simulink model "Luanvancu"  (R2018a)
settings: Solver=ode5  StartTime=0.0  StopTime=100  FixedStep=0.05  RelTol=1e-3
settings Model: PacingRate=100  Creator=Hungs  LastModifiedBy=Hungs

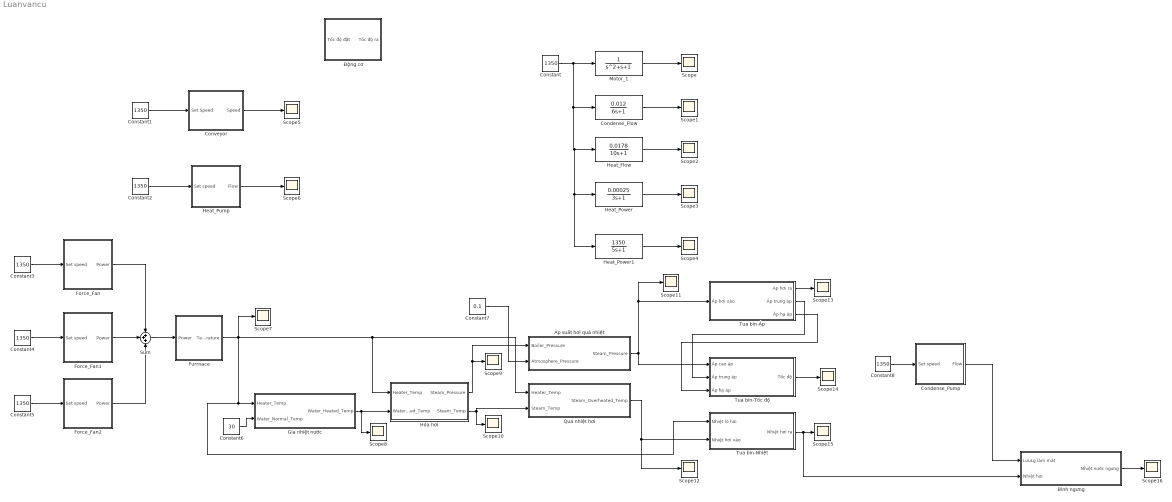
== system Luanvancu ==
  Bình ngưng : Subsystem
  Condense_Flow : TransferFcn  Numerator=[0.012]  Denominator=[6 1]
  Condense_Pump : Subsystem
      mask Display: image('C:\Program Files\MATLAB\ThermalElectricity\Maskicon\Pump.png');
  Constant{,1..5,8} (7 alike) : Constant  Value=1350
  Constant6 : Constant  Value=30
  Constant7 : Constant  Value=0.1
  Conveyor : Subsystem
      mask Display: image('C:\Program Files\MATLAB\ThermalElectricity\Maskicon\conveyor.png');
  Force_Fan : Subsystem
      mask Display: image('C:\Program Files\MATLAB\ThermalElectricity\Maskicon\Fan.png');
  Force_Fan1 : Subsystem
      mask Display: image('C:\Program Files\MATLAB\ThermalElectricity\Maskicon\Fan.png');
  Force_Fan2 : Subsystem
      mask Display: image('C:\Program Files\MATLAB\ThermalElectricity\Maskicon\Fan.png');
  Furrnace : Subsystem
      mask Display: image('C:\Program Files\MATLAB\ThermalElectricity\Maskicon\Furnace.png');
  Gia nhiệt nước : Subsystem
  Heat_Flow : TransferFcn  Numerator=[0.0178]  Denominator=[10 1]
  Heat_Power : TransferFcn  Numerator=[0.00025]  Denominator=[3 1]
  Heat_Power1 : TransferFcn  Numerator=[1350]  Denominator=[5 1]
  Heat_Pump : Subsystem
      mask Display: image('C:\Program Files\MATLAB\ThermalElectricity\Maskicon\Pump.png');
  Hóa hơi : Subsystem
  Motor_1 : TransferFcn  Denominator=[1 1 1]
  Quá nhiệt hơi : Subsystem
  Scope{,1..16} (17 alike) : Scope
  Sum : Sum  Inputs=+++
  Tua bin-Nhiệt : Subsystem
  Tua bin-Tốc độ : Subsystem
  Tua bin-Áp : Subsystem
  Áp suất hơi quá nhiệt : Subsystem
  Động cơ : Subsystem
  wires:
  Motor_1/1 -> Scope/1
  Condense_Flow/1 -> Scope1/1
  Heat_Flow/1 -> Scope2/1
  Constant/1 -> Heat_Power1/1, Heat_Power/1, Heat_Flow/1, Condense_Flow/1, Motor_1/1
  Heat_Power/1 -> Scope3/1
  Heat_Power1/1 -> Scope4/1
  Constant1/1 -> Conveyor/1(Set Speed)
  Conveyor/1(Speed) -> Scope5/1
  Constant2/1 -> Heat_Pump/1(Set speed)
  Heat_Pump/1(Flow) -> Scope6/1
  Force_Fan/1(Power) -> Sum/1
  Constant3/1 -> Force_Fan/1(Set speed)
  Furrnace/1(Temperature) -> Quá nhiệt hơi/1(Heater_Temp), Hóa hơi/1(Heater_Temp), Gia nhiệt nước/1(Heater_Temp), Tua bin-Nhiệt/1(Nhiệt lò hơi), Scope7/1
  Constant4/1 -> Force_Fan1/1(Set speed)
  Force_Fan2/1(Power) -> Sum/3
  Constant5/1 -> Force_Fan2/1(Set speed)
  Sum/1 -> Furrnace/1(Power)
  Force_Fan1/1(Power) -> Sum/2
  Constant6/1 -> Gia nhiệt nước/2(Water_Normal_Temp)
  Gia nhiệt nước/1(Water_Heated_Temp) -> Scope8/1, Hóa hơi/2(Water_Heated_Temp)
  Hóa hơi/1(Steam_Pressure) -> Áp suất hơi quá nhiệt/1(Boiler_Pressure), Scope9/1
  Hóa hơi/2(Steam_Temp) -> Quá nhiệt hơi/2(Steam_Temp), Scope10/1
  Áp suất hơi quá nhiệt/1(Steam_Pressure) -> Tua bin-Tốc độ/1(Áp cao áp), Tua bin-Áp/1(Áp hơi vào), Scope11/1
  Quá nhiệt hơi/1(Steam_Overheated_Temp) -> Tua bin-Nhiệt/2(Nhiệt hơi vào), Scope12/1
  Constant7/1 -> Áp suất hơi quá nhiệt/2(Atmosphere_Pressure)
  Tua bin-Áp/3(Áp hạ áp) -> Tua bin-Tốc độ/3(Áp hạ áp)
  Tua bin-Áp/2(Áp trung áp) -> Tua bin-Tốc độ/2(Áp trung áp)
  Tua bin-Áp/1(Áp hơi ra) -> Scope13/1
  Tua bin-Tốc độ/1(Tốc độ) -> Scope14/1
  Tua bin-Nhiệt/1(Nhiệt hơi ra) -> Bình ngưng/2(Nhiệt hơi), Scope15/1
  Constant8/1 -> Condense_Pump/1(Set speed)
  Condense_Pump/1(Flow) -> Bình ngưng/1(LưuLg làm mát)
  Bình ngưng/1(Nhiệt nước ngưng) -> Scope16/1

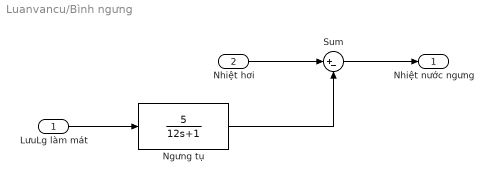
== system Luanvancu/Bình ngưng ==
  LưuLg làm mát : Inport
  Nhiệt hơi : Inport  Port=2
  Ngưng tụ : TransferFcn  Numerator=[5]  Denominator=[12 1]
  Sum : Sum  Inputs=|+-
  Nhiệt nước ngưng : Outport
  wires:
  Sum/1 -> Nhiệt nước ngưng/1
  Ngưng tụ/1 -> Sum/2
  Nhiệt hơi/1 -> Sum/1
  LưuLg làm mát/1 -> Ngưng tụ/1

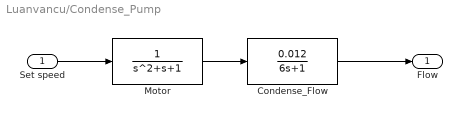
== system Luanvancu/Condense_Pump ==
  Set speed : Inport
  Condense_Flow : TransferFcn  Numerator=[0.012]  Denominator=[6 1]
  Motor : TransferFcn  Denominator=[1 1 1]
  Flow : Outport
  wires:
  Motor/1 -> Condense_Flow/1
  Set speed/1 -> Motor/1
  Condense_Flow/1 -> Flow/1

== system Luanvancu/Conveyor ==
  Set Speed : Inport
  Motor_1 : TransferFcn  Denominator=[1 1 1]
  Speed : Outport
  wires:
  Set Speed/1 -> Motor_1/1
  Motor_1/1 -> Speed/1

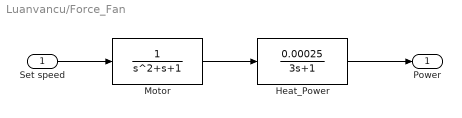
== system Luanvancu/Force_Fan ==
  Set speed : Inport
  Heat_Power : TransferFcn  Numerator=[0.00025]  Denominator=[3 1]
  Motor : TransferFcn  Denominator=[1 1 1]
  Power : Outport
  wires:
  Motor/1 -> Heat_Power/1
  Set speed/1 -> Motor/1
  Heat_Power/1 -> Power/1

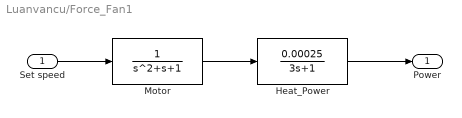
== system Luanvancu/Force_Fan1 ==
  Set speed : Inport
  Heat_Power : TransferFcn  Numerator=[0.00025]  Denominator=[3 1]
  Motor : TransferFcn  Denominator=[1 1 1]
  Power : Outport
  wires:
  Heat_Power/1 -> Power/1
  Set speed/1 -> Motor/1
  Motor/1 -> Heat_Power/1

== system Luanvancu/Force_Fan2 ==
  Set speed : Inport
  Heat_Power : TransferFcn  Numerator=[0.00025]  Denominator=[3 1]
  Motor : TransferFcn  Denominator=[1 1 1]
  Power : Outport
  wires:
  Motor/1 -> Heat_Power/1
  Set speed/1 -> Motor/1
  Heat_Power/1 -> Power/1

== system Luanvancu/Furrnace ==
  Power : Inport
  Furnace : TransferFcn  Numerator=[1350]  Denominator=[5 1]
  Temperature : Outport
  wires:
  Furnace/1 -> Temperature/1
  Power/1 -> Furnace/1

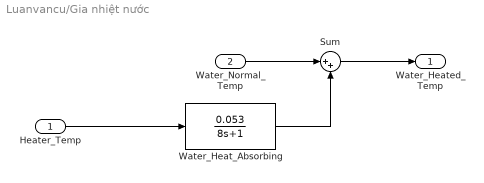
== system Luanvancu/Gia nhiệt nước ==
  Heater_Temp : Inport
  Water_Normal_Temp : Inport  Port=2
  Sum : Sum  Inputs=|++
  Water_Heat_Absorbing : TransferFcn  Numerator=[0.053]  Denominator=[8 1]
  Water_Heated_Temp : Outport
  wires:
  Heater_Temp/1 -> Water_Heat_Absorbing/1
  Water_Normal_Temp/1 -> Sum/1
  Water_Heat_Absorbing/1 -> Sum/2
  Sum/1 -> Water_Heated_Temp/1

== system Luanvancu/Heat_Pump ==
  Set speed : Inport
  Heat_Flow : TransferFcn  Numerator=[0.0178]  Denominator=[10 1]
  Motor : TransferFcn  Denominator=[1 1 1]
  Flow : Outport
  wires:
  Heat_Flow/1 -> Flow/1
  Set speed/1 -> Motor/1
  Motor/1 -> Heat_Flow/1

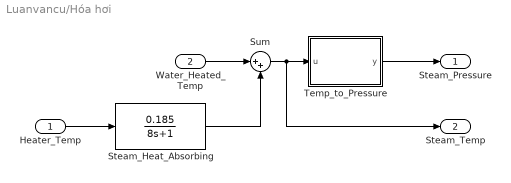
== system Luanvancu/Hóa hơi ==
  Heater_Temp : Inport
  Water_Heated_Temp : Inport  Port=2
  Steam_Heat_Absorbing : TransferFcn  Numerator=[0.185]  Denominator=[8 1]
  Sum : Sum  Inputs=|++
  Temp_to_Pressure : MATLAB Function  TreatAsAtomicUnit=on
  Steam_Pressure : Outport
  Steam_Temp : Outport  Port=2
  wires:
  Sum/1 -> Steam_Temp/1, Temp_to_Pressure/1(u)
  Steam_Heat_Absorbing/1 -> Sum/2
  Water_Heated_Temp/1 -> Sum/1
  Heater_Temp/1 -> Steam_Heat_Absorbing/1
  Temp_to_Pressure/1(y) -> Steam_Pressure/1

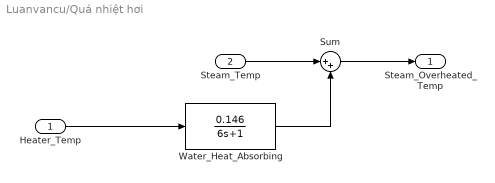
== system Luanvancu/Quá nhiệt hơi ==
  Heater_Temp : Inport
  Steam_Temp : Inport  Port=2
  Sum : Sum  Inputs=|++
  Water_Heat_Absorbing : TransferFcn  Numerator=[0.146]  Denominator=[6 1]
  Steam_Overheated_Temp : Outport
  wires:
  Sum/1 -> Steam_Overheated_Temp/1
  Water_Heat_Absorbing/1 -> Sum/2
  Steam_Temp/1 -> Sum/1
  Heater_Temp/1 -> Water_Heat_Absorbing/1

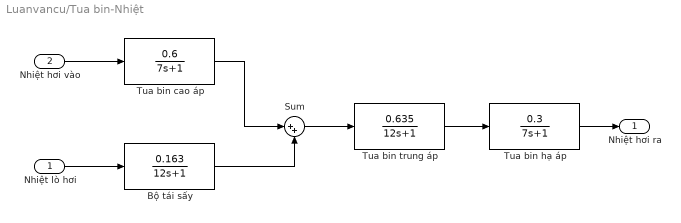
== system Luanvancu/Tua bin-Nhiệt ==
  Nhiệt lò hơi : Inport
  Nhiệt hơi vào : Inport  Port=2
  Bộ tái sấy : TransferFcn  Numerator=[0.163]  Denominator=[12 1]
  Sum : Sum  Inputs=|++
  Tua bin cao áp : TransferFcn  Numerator=[0.6]  Denominator=[7 1]
  Tua bin hạ áp : TransferFcn  Numerator=[0.3]  Denominator=[7 1]
  Tua bin trung áp : TransferFcn  Numerator=[0.635]  Denominator=[12 1]
  Nhiệt hơi ra : Outport
  wires:
  Nhiệt lò hơi/1 -> Bộ tái sấy/1
  Bộ tái sấy/1 -> Sum/2
  Nhiệt hơi vào/1 -> Tua bin cao áp/1
  Tua bin cao áp/1 -> Sum/1
  Sum/1 -> Tua bin trung áp/1
  Tua bin trung áp/1 -> Tua bin hạ áp/1
  Tua bin hạ áp/1 -> Nhiệt hơi ra/1

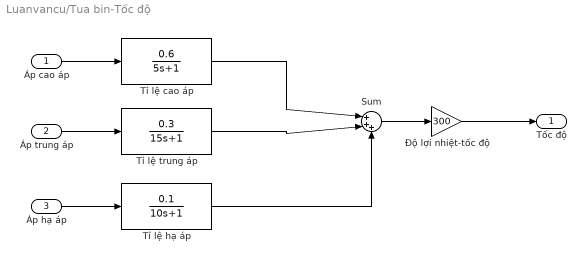
== system Luanvancu/Tua bin-Tốc độ ==
  Áp cao áp : Inport
  Áp trung áp : Inport  Port=2
  Áp hạ áp : Inport  Port=3
  Sum : Sum  Inputs=|+++
  Tỉ lệ cao áp : TransferFcn  Numerator=[0.6]  Denominator=[5 1]
  Tỉ lệ hạ áp : TransferFcn  Numerator=[0.1]  Denominator=[10 1]
  Tỉ lệ trung áp : TransferFcn  Numerator=[0.3]  Denominator=[15 1]
  Độ lợi nhiệt-tốc độ : Gain  Gain=300
  Tốc độ : Outport
  wires:
  Áp cao áp/1 -> Tỉ lệ cao áp/1
  Tỉ lệ cao áp/1 -> Sum/1
  Sum/1 -> Độ lợi nhiệt-tốc độ/1
  Áp trung áp/1 -> Tỉ lệ trung áp/1
  Áp hạ áp/1 -> Tỉ lệ hạ áp/1
  Tỉ lệ trung áp/1 -> Sum/2
  Tỉ lệ hạ áp/1 -> Sum/3
  Độ lợi nhiệt-tốc độ/1 -> Tốc độ/1

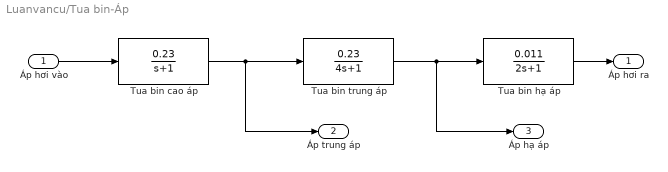
== system Luanvancu/Tua bin-Áp ==
  Áp hơi vào : Inport
  Tua bin cao áp : TransferFcn  Numerator=[0.23]  Denominator=[1 1]
  Tua bin hạ áp : TransferFcn  Numerator=[0.011]  Denominator=[2 1]
  Tua bin trung áp : TransferFcn  Numerator=[0.23]  Denominator=[4 1]
  Áp hơi ra : Outport
  Áp trung áp : Outport  Port=2
  Áp hạ áp : Outport  Port=3
  wires:
  Tua bin hạ áp/1 -> Áp hơi ra/1
  Tua bin trung áp/1 -> Áp hạ áp/1, Tua bin hạ áp/1
  Tua bin cao áp/1 -> Áp trung áp/1, Tua bin trung áp/1
  Áp hơi vào/1 -> Tua bin cao áp/1

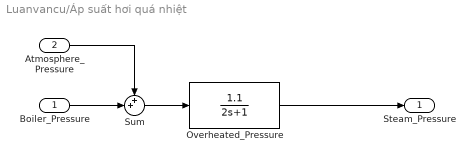
== system Luanvancu/Áp suất hơi quá nhiệt ==
  Boiler_Pressure : Inport
  Atmosphere_Pressure : Inport  Port=2
  Overheated_Pressure : TransferFcn  Numerator=[1.1]  Denominator=[2 1]
  Sum : Sum  Inputs=++|
  Steam_Pressure : Outport
  wires:
  Overheated_Pressure/1 -> Steam_Pressure/1
  Boiler_Pressure/1 -> Sum/2
  Sum/1 -> Overheated_Pressure/1
  Atmosphere_Pressure/1 -> Sum/1

== system Luanvancu/Động cơ ==
  Tốc độ đặt : Inport
  Bão hòa 2 cực : Saturate  UpperLimit=1500  LowerLimit=0
  Động cơ AC : TransferFcn  Denominator=[1 1 1]
  Tốc độ ra : Outport
  wires:
  Bão hòa 2 cực/1 -> Tốc độ ra/1
  Tốc độ đặt/1 -> Động cơ AC/1
  Động cơ AC/1 -> Bão hòa 2 cực/1

== matlab function Luanvancu/Hóa hơi/Temp_to_Pressure ==
  data: u input; y output
function y = fcn(u)
to = [29.95 32.89 41.53 45.82 52.57 60.08 69.12 75.87 81.33 93.5 99.62 109.32 ...
    120.24 133.56 143.64 151.87 158.86 164.98 170.44 175.39 179.92 195.08 212.42 ...
    233.89 250.39 263.98 285.86 311.03 342.34 357.04 365.80 373.70];
p = [0.004 0.005 0.008 0.01 0.018 0.02 0.03 0.04 0.05 0.08 0.1 0.14 0.2 0.3 0.4 ...
    0.5 0.6 0.7 0.8 0.9 1 1.4 2 3 4 5 7 10 15 18 20 22];
y = interp1(to,p,u);
